simulink library "ilcPhase_cl"  (R2018b)
settings: Solver=VariableStepAuto  StartTime=0.0  StopTime=10.0  RelTol=1e-3
libraries: simulink x7, stopwatch_ul x1
settings Model: Creator=mcobb  LastModifiedBy=mcobb

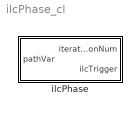
== system ilcPhase_cl ==
  ilcPhase : Subsystem  TreatAsAtomicUnit=on  mask{upperLim=0, lowerLim=0, numInitLaps=0}
      mask prompts: upperLim "Upper Limit"; lowerLim "Lower Limit"; numInitLaps "Num Initialization Laps"
      settings: MinAlgLoopOccurrences=on

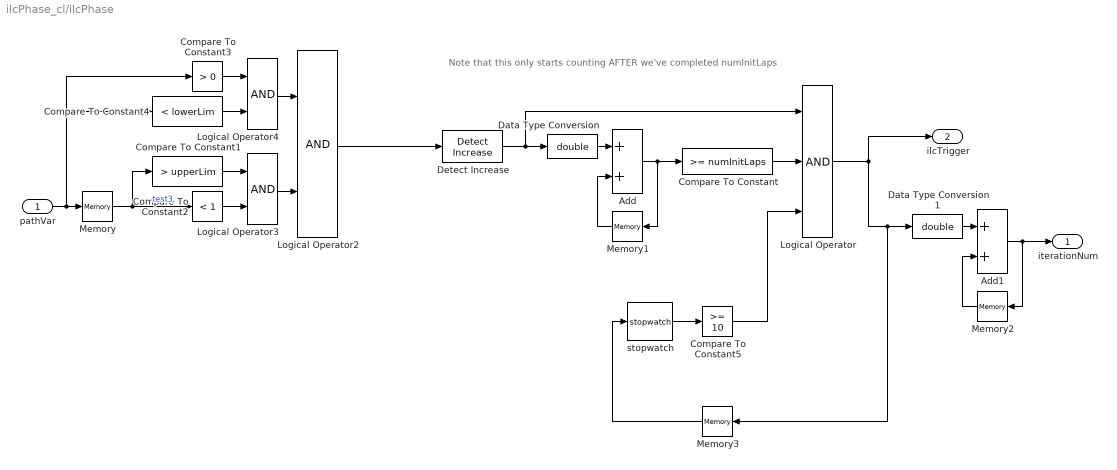
== system ilcPhase_cl/ilcPhase ==
  note: Note that this only starts counting AFTER we've completed numInitLaps
  pathVar : Inport
  Add : Sum
  Add1 : Sum
  Compare To Constant : simulink/Logic and Bit Operations/Compare To Constant  relop=>=  const=numInitLaps  OutDataTypeStr=boolean
  Compare To Constant1 : simulink/Logic and Bit Operations/Compare To Constant  relop=>  const=upperLim  OutDataTypeStr=boolean
  Compare To Constant2 : simulink/Logic and Bit Operations/Compare To Constant  relop=<  const=1  OutDataTypeStr=boolean
  Compare To Constant3 : simulink/Logic and Bit Operations/Compare To Constant  relop=>  const=0  OutDataTypeStr=boolean
  Compare To Constant4 : simulink/Logic and Bit Operations/Compare To Constant  relop=<  const=lowerLim  OutDataTypeStr=boolean
  Compare To Constant5 : simulink/Logic and Bit Operations/Compare To Constant  relop=>=  const=10  OutDataTypeStr=boolean
  Data Type Conversion : DataTypeConversion  OutDataTypeStr=double
  Data Type Conversion1 : DataTypeConversion  OutDataTypeStr=double
  Detect Increase : simulink/Logic and Bit Operations/Detect Increase  vinit=0.0  OutDataTypeStr=boolean
  Logical Operator : Logic  Inputs=3  AllPortsSameDT=off  OutDataTypeStr=boolean
  Logical Operator2 : Logic  AllPortsSameDT=off  OutDataTypeStr=boolean
  Logical Operator3 : Logic  AllPortsSameDT=off  OutDataTypeStr=boolean
  Logical Operator4 : Logic  AllPortsSameDT=off  OutDataTypeStr=boolean
  Memory : Memory  InheritSampleTime=on
  Memory1 : Memory  InheritSampleTime=on
  Memory2 : Memory  InheritSampleTime=on
  Memory3 : Memory  InitialCondition=false
  stopwatch : stopwatch_ul/stopwatch  SystemSampleTime=-1
  iterationNum : Outport
  ilcTrigger : Outport  Port=2
  wires:
  pathVar/1 -> Memory/1, Compare To Constant3/1, Compare To Constant4/1
  Data Type Conversion/1 -> Add/1
  Memory1/1 -> Add/2
  Detect Increase/1 -> Logical Operator/1, Data Type Conversion/1
  Add/1 -> Compare To Constant/1, Memory1/1
  Logical Operator2/1 -> Detect Increase/1
  Logical Operator3/1 -> Logical Operator2/2
  Compare To Constant2/1 -> Logical Operator3/2
  Compare To Constant1/1 -> Logical Operator3/1
  Logical Operator4/1 -> Logical Operator2/1
  Compare To Constant3/1 -> Logical Operator4/1
  Compare To Constant4/1 -> Logical Operator4/2
  Memory/1 -> Compare To Constant1/1, Compare To Constant2/1  "test3"
  Compare To Constant/1 -> Logical Operator/2
  Logical Operator/1 -> ilcTrigger/1, Memory3/1, Data Type Conversion1/1
  Add1/1 -> iterationNum/1, Memory2/1
  Memory2/1 -> Add1/2
  Data Type Conversion1/1 -> Add1/1
  Memory3/1 -> stopwatch/1
  stopwatch/1 -> Compare To Constant5/1
  Compare To Constant5/1 -> Logical Operator/3
